simulink model "Testfunktion44b"  (R2017a)
settings: Solver=VariableStepAuto  StartTime=0.0  StopTime=10.0  RelTol=1e-3
libraries: cstblocks x1
settings Model: Creator=prt01  LastModifiedBy=prt01

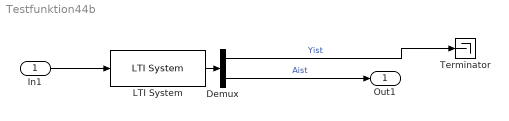
== system Testfunktion44b ==
  In1 : Inport
  Demux : Demux  Outputs=2
  LTI System : cstblocks/LTI System  sys=test  IC=[]
  Terminator : Terminator
  Out1 : Outport
  wires:
  Demux/2 -> Out1/1  "Aist"
  LTI System/1 -> Demux/1
  Demux/1 -> Terminator/1  "Yist"
  In1/1 -> LTI System/1
